simulink model "MicroADPCPU2"  (R2024a)
settings: Solver=FixedStepAuto  StartTime=0.0  StopTime=Inf  RelTol=1e-3  EnableMultiTasking=on
values from neighbouring files (symbols this model uses):
  PI_params = mcb.internal.SetControllerParameters(pmsm,inverter,SI_System,T_pwm,Ts,Ts_speed)    [Para_Motor_Micro.m]
  Ts = T_pwm    (= 3e-05)    [Para_Motor_Micro.m]
  Ts_speed = 10*1*Ts    (= 0.0003)    [Para_Motor_Micro.m]
undefined symbols (not defined in the file or in its folder): C28x, CPU1, CPU2, DiscIntNeverNeededParam
libraries: c2837xDlib x6, mcbcontrolslib x2, c280xlib x2, c2000lib x1, slpidlib x1, svdutilitieslib x1, simulink x1
settings Model: ExtModeTrigDuration=8  Creator=axel_  LastModifiedBy=axel_
settings SolverCC: AutoInsertRateTranBlk=on
settings OptimizationCC: DefaultParameterBehavior=Inlined  DefaultUnderspecifiedDataType=single  EnhancedBackFolding=on  PassReuseOutputArgsAs=Individual arguments  MaxStackSize=1024  OptimizeBlockOrder=speed  DifferentSizesBufferReuse=on  OptimizationCustomize=off  DenormalBehavior=FlushToZero  EfficientTunableParamExpr=on
settings DebuggingCC: MultiTaskDSMMsg=none  ParameterPrecisionLossMsg=none  ParameterTunabilityLossMsg=error
settings HardwareCC: ProdBitPerChar=16  ProdBitPerInt=16  ProdBitPerPointer=32  ProdBitPerSizeT=32  ProdBitPerPtrDiffT=32  ProdLargestAtomicInteger=Integer  ProdLargestAtomicFloat=None  ProdWordSize=16  ProdLongLongMode=on  ProdHWDeviceType=Texas Instruments->C2000
settings ModelReferenceCC: ModelReferenceNumInstancesAllowed=Single
settings SFSimCC: MATLABDynamicMemAlloc=off
settings RTWCC: Description=Embedded Coder  SystemTargetFile=ert.tlc  HardwareBoard=TI Delfino F2837xD  TemplateMakefile=ert_default_tmf  Toolchain=Texas Instruments Code Composer Studio (C2000)  CodeProfilingSaveOptions=MetricsOnly  GPUComputeCapability=3.5
settings CodeAppCC: ForceParamTrailComments=on  IgnoreCustomStorageClasses=off  OperatorAnnotations=on  SimulinkDataObjDesc=on  SFDataObjDesc=on  InsertBlockDesc=on
settings ERTTargetCC: CodeReplacementLibrary=TI C28x  ExtModeTransport=4  ExtModeStaticAlloc=on  ExtModeAutomaticAllocSize=off  ExtModeStaticAllocSize=10000  ExtModeMexFile=ext_xcp  ExtModeIntrfLevel=Level2 - Open  InlinedParameterPlacement=NonHierarchical

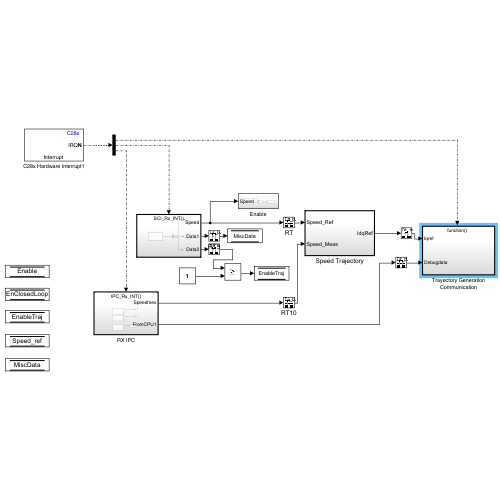
[thumbnail: Simulink's stored preview of the top-level diagram]
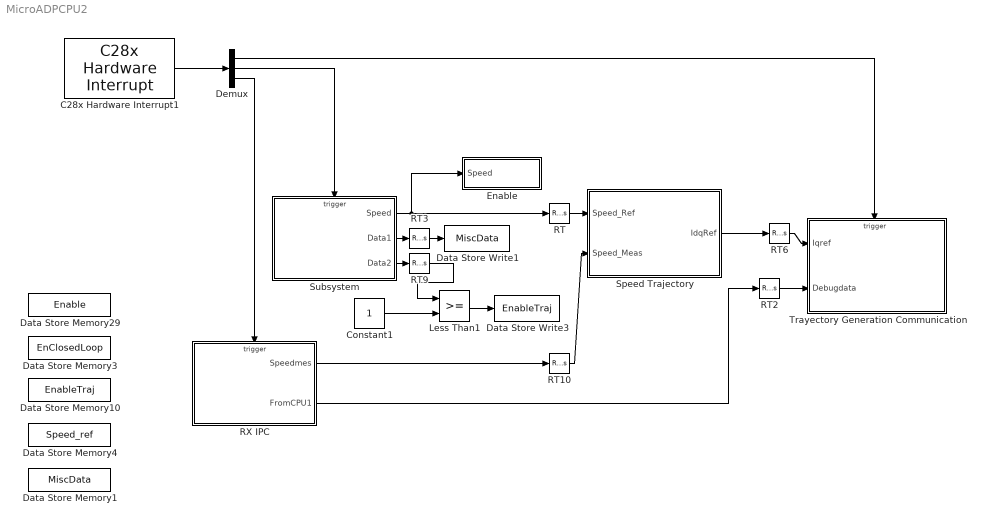
== system MicroADPCPU2 ==
  C28x Hardware Interrupt1 : c2000lib/Scheduling/C28x Hardware Interrupt  irqnumbers=[1 9 1]  pienumbers=[1 1 13]  irqpriorities="[30 50  31]"  irqpreempts=[1 0 1 ]  showinput=off  dspchiptype=C280X
  Constant1 : Constant
  Data Store Memory1 : DataStoreMemory  DataStoreName=MiscData  ShowAdditionalParam=off  OutDataTypeStr=single
  Data Store Memory10 : DataStoreMemory  DataStoreName=EnableTraj  ShowAdditionalParam=off  OutDataTypeStr=boolean
  Data Store Memory29 : DataStoreMemory  DataStoreName=Enable  ShowAdditionalParam=off  OutDataTypeStr=boolean
  Data Store Memory3 : DataStoreMemory  DataStoreName=EnClosedLoop  ShowAdditionalParam=off  OutDataTypeStr=boolean
  Data Store Memory4 : DataStoreMemory  DataStoreName=Speed_ref  InitialValue=20  ShowAdditionalParam=off  OutDataTypeStr=single
  Data Store Write1 : DataStoreWrite  DataStoreName=MiscData  IndexOptions=Index vector (dialog)  Indices=1  OutputSizes=1
  Data Store Write3 : DataStoreWrite  DataStoreName=EnableTraj  IndexOptions=Index vector (dialog)  Indices=1  OutputSizes=1
  Demux : Demux  Outputs=3
  Enable : Subsystem
  Less Than1 : RelationalOperator  OutDataTypeStr=boolean  RndMeth=Simplest  InputSameDT=off
  RT : RateTransition  Deterministic=off  OutPortSampleTime=Ts_speed
  RT10 : RateTransition  Deterministic=off  OutPortSampleTime=Ts_speed
  RT{2..3,6,9} (4 alike) : RateTransition  Deterministic=off
  RX IPC : Subsystem
  Speed Trajectory : Subsystem  TreatAsAtomicUnit=on  SystemSampleTime=Ts_speed
  Subsystem : Subsystem
  Trayectory Generation Communication : Subsystem  TreatAsAtomicUnit=on
  wires:
  C28x Hardware Interrupt1/1 -> Demux/1
  Demux/1 -> Trayectory Generation Communication/Trigger
  Constant1/1 -> Less Than1/2
  Less Than1/1 -> Data Store Write3/1
  Speed Trajectory/1(IdqRef) -> RT6/1
  RT3/1 -> Data Store Write1/1
  RT10/1 -> Speed Trajectory/2(Speed_Meas)
  Subsystem/1(Speed) -> Enable/1(Speed), RT/1
  Subsystem/3(Data2) -> RT9/1
  RT9/1 -> Less Than1/1
  Subsystem/2(Data1) -> RT3/1
  RT/1 -> Speed Trajectory/1(Speed_Ref)
  Demux/2 -> Subsystem/Trigger
  Demux/3 -> RX IPC/Trigger
  RX IPC/1(Speedmes) -> RT10/1
  RT6/1 -> Trayectory Generation Communication/1(Iqref)
  RX IPC/2(FromCPU1) -> RT2/1
  RT2/1 -> Trayectory Generation Communication/2(Debugdata)

== system MicroADPCPU2/Enable ==
  Speed : Inport
  Constant1 : Constant  Value=0
  Data Store Write : DataStoreWrite  DataStoreName=Enable  IndexOptions=Index vector (dialog)  Indices=1  OutputSizes=1
  Less Than : RelationalOperator  Operator=~=  OutDataTypeStr=boolean  RndMeth=Simplest  InputSameDT=off
  wires:
  Less Than/1 -> Data Store Write/1
  Constant1/1 -> Less Than/2
  Speed/1 -> Less Than/1

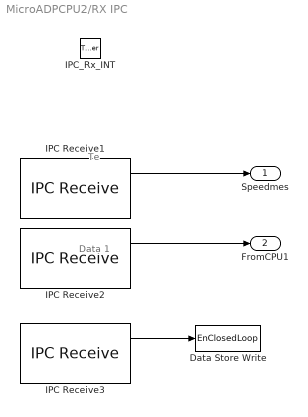
== system MicroADPCPU2/RX IPC ==
  note: Data 1
  note: Te
  IPC_Rx_INT : TriggerPort  TriggerType=function-call  VariantControl=Variant
  Data Store Write : DataStoreWrite  DataStoreName=EnClosedLoop  IndexOptions=Index vector (dialog)  Indices=1  OutputSizes=1
  IPC Receive1 : c2837xDlib/IPC Receive  blkParamProc=F2837x  SelectSource=C28x (CPU1/CPU2)  SelectChannel=0  DataType=single  DataLength=1  EnableBlocking=off  SampleTime=-1
  IPC Receive2 : c2837xDlib/IPC Receive  blkParamProc=F2837x  SelectSource=C28x (CPU1/CPU2)  SelectChannel=1  DataType=single  DataLength=2  EnableBlocking=off  SampleTime=-1
  IPC Receive3 : c2837xDlib/IPC Receive  blkParamProc=F2837x  SelectSource=C28x (CPU1/CPU2)  SelectChannel=4  DataType=boolean  DataLength=1  EnableBlocking=off  SampleTime=-1
  Speedmes : Outport
  FromCPU1 : Outport  Port=2
  wires:
  IPC Receive1/1 -> Speedmes/1
  IPC Receive2/1 -> FromCPU1/1
  IPC Receive3/1 -> Data Store Write/1

== system MicroADPCPU2/Speed Trajectory ==
  Speed_Ref : Inport
  Speed_Meas : Inport  Port=2
  PI_Controller_Speed : Subsystem
  Subsystem : Subsystem
  IdqRef : Outport  VectorParamsAs1DForOutWhenUnconnected=off
  wires:
  Speed_Meas/1 -> PI_Controller_Speed/2(N_fb), Subsystem/2(Speed_Ref_Open)  "Speed_fb"
  Speed_Ref/1 -> Subsystem/1(Speed_Ref_In)
  Subsystem/1(Speed_Ref_PU) -> IdqRef/1, PI_Controller_Speed/1(N_ref)  "Speed_Ref"

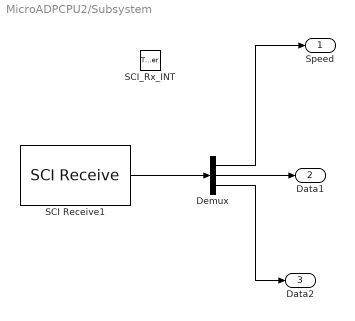
== system MicroADPCPU2/Subsystem ==
  SCI_Rx_INT : TriggerPort  TriggerType=function-call  VariantControl=Variant
  Demux : Demux  Outputs=3
  SCI Receive1 : c280xlib/SCI Receive  sciModule=A  dataHead=''  headerCheckMaxCount=16  dataTail=''  dataType=single  dataLenOptions=Length via dialog  dataDim=3  maxDataLength=1  initValue=0  errOption=Output the last received value  errValue=0  sampleTime=-1  blockingMode=on  timeOut=0.00875  outputStatus=off
  Speed : Outport
  Data1 : Outport  Port=2
  Data2 : Outport  Port=3
  wires:
  Demux/2 -> Data1/1
  SCI Receive1/1 -> Demux/1
  Demux/1 -> Speed/1
  Demux/3 -> Data2/1

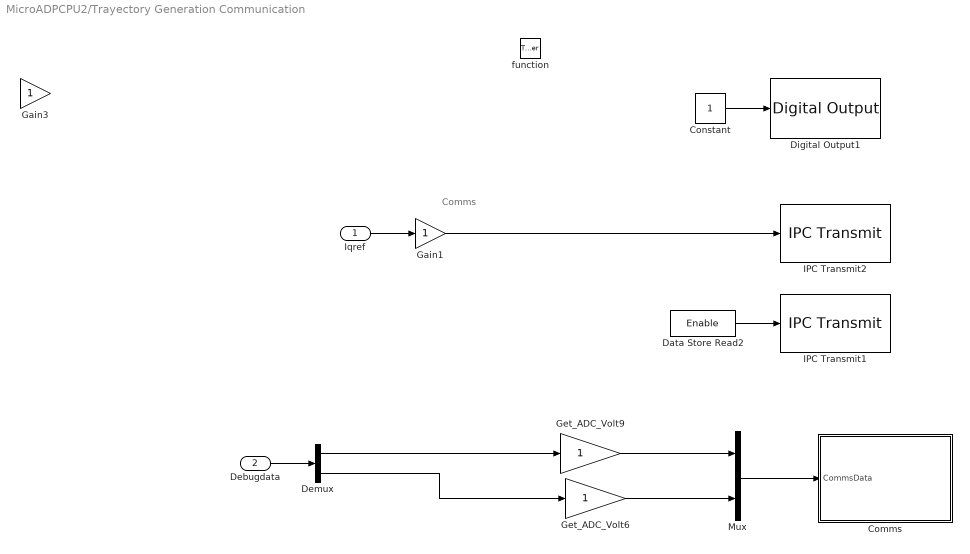
== system MicroADPCPU2/Trayectory Generation Communication ==
  note: Comms
  Iqref : Inport
  Debugdata : Inport  Port=2
  function : TriggerPort  TriggerType=function-call  VariantControl=Variant  OutputDataType=int8
  Comms : Subsystem  SystemSampleTime=5e-5
  Constant : Constant
  Data Store Read2 : DataStoreRead  DataStoreName=Enable  IndexOptions=Index vector (dialog)  Indices=1  OutputSizes=1
  Demux : Demux  Outputs=2
  Digital Output1 : c2837xDlib/Digital Output  GPIO_Number=GPIO16~GPIO23  GPIO_Bit0=off  GPIO_BIT0_Toggle=on  GPIO_Bit1=off  GPIO_BIT1_Toggle=off  GPIO_Bit2=off  GPIO_BIT2_Toggle=off  GPIO_Bit3=off  GPIO_BIT3_Toggle=off  GPIO_Bit4=off  GPIO_BIT4_Toggle=off  GPIO_Bit5=off  GPIO_BIT5_Toggle=off  GPIO_Bit6=on  GPIO_BIT6_Toggle=on  GPIO_Bit7=off  GPIO_BIT7_Toggle=off
  Gain1 : Gain  OutDataTypeStr=single
  Gain3 : Gain  OutDataTypeStr=single
  Get_ADC_Volt6 : Gain  OutDataTypeStr=single  RndMeth=Simplest
  Get_ADC_Volt9 : Gain  OutDataTypeStr=single  RndMeth=Simplest
  IPC Transmit1 : c2837xDlib/IPC Transmit  blkParamProc=F2837x  SelectDestination=C28x (CPU1/CPU2)  SelectChannel=3  EnableBlocking=off
  IPC Transmit2 : c2837xDlib/IPC Transmit  blkParamProc=F2837x  SelectDestination=C28x (CPU1/CPU2)  SelectChannel=2  EnableBlocking=off
  Mux : Mux  Inputs=2
  wires:
  Get_ADC_Volt9/1 -> Mux/1
  Get_ADC_Volt6/1 -> Mux/2
  Mux/1 -> Comms/1(CommsData)
  Data Store Read2/1 -> IPC Transmit1/1
  Iqref/1 -> Gain1/1
  Debugdata/1 -> Demux/1
  Gain1/1 -> IPC Transmit2/1
  Constant/1 -> Digital Output1/1
  Demux/1 -> Get_ADC_Volt9/1
  Demux/2 -> Get_ADC_Volt6/1

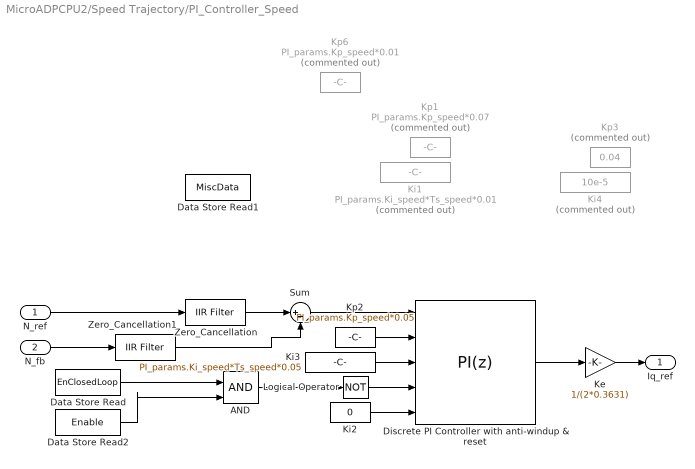
== system MicroADPCPU2/Speed Trajectory/PI_Controller_Speed ==
  N_ref : Inport
  N_fb : Inport  Port=2
  AND : Logic  IconShape=distinctive  AllPortsSameDT=off  OutDataTypeStr=boolean
  Data Store Read : DataStoreRead  DataStoreName=EnClosedLoop  IndexOptions=Index vector (dialog)  Indices=1  OutputSizes=1
  Data Store Read1 : DataStoreRead  DataStoreName=MiscData  IndexOptions=Index vector (dialog)  Indices=1  OutputSizes=1
  Data Store Read2 : DataStoreRead  DataStoreName=Enable  IndexOptions=Index vector (dialog)  Indices=1  OutputSizes=1
  Discrete PI Controller with anti-windup & reset : slpidlib/PID Controller  Controller=PI  Form=Parallel  TimeDomain=Discrete-time  UseExternalTs=off  SampleTime=-1  IntegratorMethod=Forward Euler  FilterMethod=Forward Euler  ControllerParametersSource=external  P=1  I=1  UseKiTs=on  D=0  UseExternalDerivativeSource=off  N=100  UseFilter=on  TunerSelectOption=Transfer Function Based (PID Tuner App)  InitialConditionSource=external  InitialConditionForIntegrator=0  InitialConditionForFilter=0  DifferentiatorICPrevScaledInput=0  ExternalReset=level  TrackingMode=off  Kt=1  LimitOutput=on  SatLimitsSource=internal  UpperSaturationLimit=3.5  LowerSaturationLimit=-3.5  LinearizeAsGain=on  AntiWindupMode=clamping  Kb=1  LimitIntegrator=off  UpperIntegratorSaturationLimit=inf  LowerIntegratorSaturationLimit=-inf  RndMeth=Simplest  POutMin=[]  POutMax=[]  IOutMin=[]  IOutMax=[]  DOutMin=[]  DOutMax=[]  NOutMin=[]  NOutMax=[]  SumOutMin=[]  SumOutMax=[]  SaturationOutDataTypeStr=Inherit: Inherit via back propagation  SaturationOutMin=[]  SaturationOutMax=[]  PParamMin=[]  PParamMax=[]  IParamMin=[]  IParamMax=[]  DParamMin=[]  DParamMax=[]  NParamMin=[]  NParamMax=[]  KbParamMin=[]  KbParamMax=[]  KtParamMin=[]  KtParamMax=[]  KbOutMin=[]  KbOutMax=[]  KtOutMin=[]  KtOutMax=[]  IntegratorOutMin=[]  IntegratorOutMax=[]  FilterOutMin=[]  FilterOutMax=[]  SumI1OutMin=[]  SumI1OutMax=[]  SumI2OutMin=[]  SumI2OutMax=[]  SumI3OutMin=[]  SumI3OutMax=[]  SumI4OutMin=[]  SumI4OutMax=[]  SumDOutMin=[]  SumDOutMax=[]  DifferentiatorOutMin=[]  DifferentiatorOutMax=[]  FilterDiffOutCoefMin=[]  FilterDiffOutCoefMax=[]  ReciprocalOutMin=[]  ReciprocalOutMax=[]  SumDenOutMin=[]  SumDenOutMax=[]  SumNumOutMin=[]  SumNumOutMax=[]  DivideOutMin=[]  DivideOutMax=[]  UdiffTsProdOutMin=[]  UdiffTsProdOutMax=[]  NTsProdOutMin=[]  NTsProdOutMax=[]  UintegralTsProdOutMin=[]  UintegralTsProdOutMax=[]  UngainTsProdOutMin=[]  UngainTsProdOutMax=[]  ClampingZeroOutDataTypeStr=Inherit: Inherit via back propagation  ClampingZeroOutMin=[]  ClampingZeroOutMax=[]  FilterDenConstantOutDataTypeStr=Inherit: Inherit via back propagation  FilterDenConstantOutMin=[]  FilterDenConstantOutMax=[]  PCopyOutDataTypeStr=Inherit: Inherit via back propagation  PCopyOutMin=[]  PCopyOutMax=[]  NCopyOutDataTypeStr=Inherit: Inherit via back propagation  NCopyOutMin=[]  NCopyOutMax=[]  IntegratorContinuousStateAttributes=''  IntegratorStateMustResolveToSignalObject=off  IntegratorRTWStateStorageClass=Auto  FilterContinuousStateAttributes=''  FilterStateMustResolveToSignalObject=off  FilterRTWStateStorageClass=Auto  ParallelPVariant=ExternalParameters  IdealPVariant=Disabled  IVariant=ExternalParameters  DVariant=Disabled  IntegratorVariant=Discrete  SatVariant=Enabled  AWVariant=DiscClampingParallel  PCopyVariant=Disabled  TRVariant=Disabled  FdbkBlocksVariant=Forward  IdealPFdbkVariant=Disabled  SatFdbkVariant=Disabled  DerivativeFilterVariant=Disabled  NVariant=Disabled  NCopyVariant=Disabled_SignalSpec  FilterICVariant=Disabled  IntegratorICVariant=ExternalICs  ExternalResetVariant=ExternalReset  TRSumVariant=Passthrough  SumFdbkVariant=Disabled  SumVariant=Sum_PI  TsampFilterVariant=InternalTs  TsampNgainVariant=Passthrough  TsampIntegralVariant=Disabled_SignalSpec  ExternalSaturationOutDataTypeStr=Inherit: Same as second input  DerivativeSourceVariant=Disabled
      settings: LibrarySourceBlock=mcbcontrolslib/PI Controller
  Ke : Gain  Gain=1/(2*0.3631)  OutDataTypeStr=single
  Ki1 : Constant  Commented=on  Value=PI_params.Ki_speed*Ts_speed*0.01  OutDataTypeStr=double  SampleTime=-1
  Ki2 : Constant  Value=0  OutDataTypeStr=dataType  SampleTime=-1
  Ki3 : Constant  Value=PI_params.Ki_speed*Ts_speed*0.05  OutDataTypeStr=double  SampleTime=-1
  Ki4 : Constant  Commented=on  Value=10e-5  OutDataTypeStr=double  SampleTime=-1
  Kp1 : Constant  Commented=on  Value=PI_params.Kp_speed*0.07  OutDataTypeStr=double  SampleTime=-1
  Kp2 : Constant  Value=PI_params.Kp_speed*0.05  OutDataTypeStr=double  SampleTime=-1
  Kp3 : Constant  Commented=on  Value=0.04  OutDataTypeStr=double  SampleTime=-1
  Kp6 : Constant  Commented=on  Value=PI_params.Kp_speed*0.01  OutDataTypeStr=double  SampleTime=-1
  Logical Operator : Logic  Operator=NOT  IconShape=distinctive  AllPortsSameDT=off  OutDataTypeStr=boolean
  Sum : Sum  Inputs=|+-  OutDataTypeStr=Inherit: Same as first input
  Zero_Cancellation : mcbcontrolslib/IIR Filter  VariantControl=Low Pass Filter  VariantSelect=Low-pass  FilterConstantInputType=Specify via dialog  Filter_constant=0.01*(Ts_speed/Ts)  advancedSettings=off  Ts=50e-6  cutOff_freq=353.6777
  Zero_Cancellation1 : mcbcontrolslib/IIR Filter  VariantControl=Low Pass Filter  VariantSelect=Low-pass  FilterConstantInputType=Specify via dialog  Filter_constant=0.01*(Ts_speed/Ts)  advancedSettings=off  Ts=50e-6  cutOff_freq=353.6777
  Iq_ref : Outport  VectorParamsAs1DForOutWhenUnconnected=off
  wires:
  Discrete PI Controller with anti-windup & reset/1 -> Ke/1
  Sum/1 -> Discrete PI Controller with anti-windup & reset/1
  Logical Operator/1 -> Discrete PI Controller with anti-windup & reset/4
  Ki2/1 -> Discrete PI Controller with anti-windup & reset/5
  AND/1 -> Logical Operator/1
  N_ref/1 -> Zero_Cancellation/1
  N_fb/1 -> Zero_Cancellation1/1
  Zero_Cancellation/1 -> Sum/1
  Data Store Read/1 -> AND/1
  Data Store Read2/1 -> AND/2
  Ki3/1 -> Discrete PI Controller with anti-windup & reset/3
  Kp2/1 -> Discrete PI Controller with anti-windup & reset/2
  Zero_Cancellation1/1 -> Sum/2
  Ke/1 -> Iq_ref/1

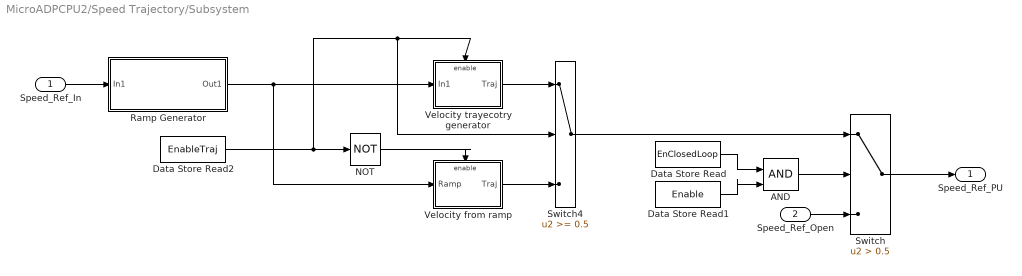
== system MicroADPCPU2/Speed Trajectory/Subsystem ==
  Speed_Ref_In : Inport
  Speed_Ref_Open : Inport  Port=2
  AND : Logic  IconShape=distinctive  AllPortsSameDT=off  OutDataTypeStr=boolean
  Data Store Read : DataStoreRead  DataStoreName=EnClosedLoop  IndexOptions=Index vector (dialog)  Indices=1  OutputSizes=1
  Data Store Read1 : DataStoreRead  DataStoreName=Enable  IndexOptions=Index vector (dialog)  Indices=1  OutputSizes=1
  Data Store Read2 : DataStoreRead  DataStoreName=EnableTraj  IndexOptions=Index vector (dialog)  Indices=1  OutputSizes=1
  NOT : Logic  Operator=NOT  IconShape=distinctive  AllPortsSameDT=off  OutDataTypeStr=boolean
  Ramp Generator : Subsystem
  Switch : Switch  Criteria=u2 > Threshold  Threshold=0.5  SaturateOnIntegerOverflow=off  InputSameDT=off
  Switch4 : Switch  Threshold=0.5  OutDataTypeStr=Inherit: Inherit via back propagation  RndMeth=Simplest  SaturateOnIntegerOverflow=off  InputSameDT=off
  Velocity from ramp : Subsystem
  Velocity trayecotry generator : Subsystem
  Speed_Ref_PU : Outport
  wires:
  Switch/1 -> Speed_Ref_PU/1
  Speed_Ref_Open/1 -> Switch/3
  AND/1 -> Switch/2
  Data Store Read/1 -> AND/1
  Data Store Read1/1 -> AND/2
  Data Store Read2/1 -> Switch4/2, Velocity trayecotry generator/Enable, NOT/1
  Velocity from ramp/1(Traj) -> Switch4/3
  NOT/1 -> Velocity from ramp/Enable
  Velocity trayecotry generator/1(Traj) -> Switch4/1
  Switch4/1 -> Switch/1
  Ramp Generator/1(Out1) -> Velocity trayecotry generator/1(In1), Velocity from ramp/1(Ramp)
  Speed_Ref_In/1 -> Ramp Generator/1(In1)

== system MicroADPCPU2/Trayectory Generation Communication/Comms ==
  CommsData : Inport
  SCI (Serial Comunication) : Subsystem
  Selector : Selector  InputPortWidth=2  IndexOptions=Index vector (port)  Indices=[1 3]  OutputSizes=1
  speed_control : Constant  Value=[1 2]  OutDataTypeStr=uint16  SampleTime=-1
  wires:
  Selector/1 -> SCI (Serial Comunication)/1(In1)
  CommsData/1 -> Selector/1
  speed_control/1 -> Selector/2

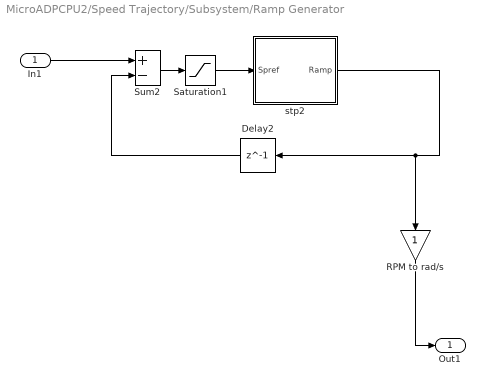
== system MicroADPCPU2/Speed Trajectory/Subsystem/Ramp Generator ==
  In1 : Inport
  Delay2 : Delay  DelayLength=1
  RPM to rad/s : Gain  OutDataTypeStr=single  RndMeth=Simplest
  Saturation1 : Saturate  UpperLimit=2.5e-3  LowerLimit=-2.5e-3  OutDataTypeStr=double
  Sum2 : Sum  Inputs=+-
  stp2 : MATLAB Function  TreatAsAtomicUnit=on
  Out1 : Outport
  wires:
  Saturation1/1 -> stp2/1(Spref)
  stp2/1(Ramp) -> RPM to rad/s/1, Delay2/1
  Delay2/1 -> Sum2/2
  RPM to rad/s/1 -> Out1/1
  Sum2/1 -> Saturation1/1
  In1/1 -> Sum2/1

== system MicroADPCPU2/Speed Trajectory/Subsystem/Velocity from ramp ==
  Ramp : Inport
  Enable : EnablePort  StatesWhenEnabling=reset
  Traj : Outport  VectorParamsAs1DForOutWhenUnconnected=off
  wires:
  Ramp/1 -> Traj/1

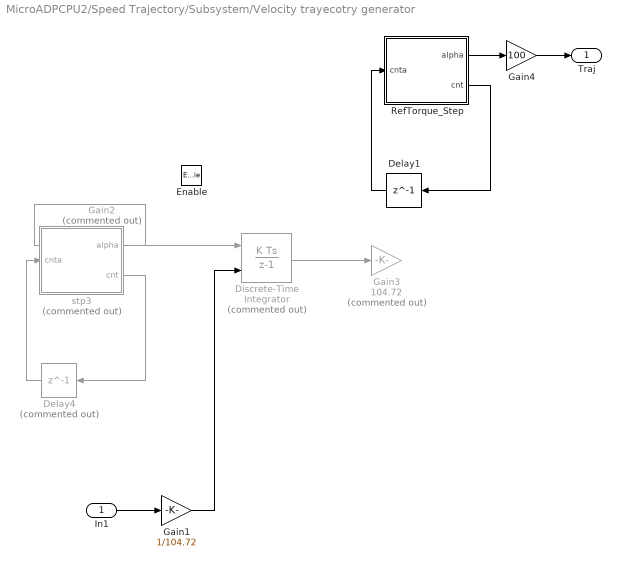
== system MicroADPCPU2/Speed Trajectory/Subsystem/Velocity trayecotry generator ==
  In1 : Inport
  Enable : EnablePort  StatesWhenEnabling=reset
  Delay1 : Delay  DelayLength=1
  Delay4 : Delay  Commented=on  DelayLength=1
  Discrete-Time Integrator : DiscreteIntegrator  Commented=on  InitialConditionSource=external  InitialCondition=0.47746371  SampleTime=-1  ICPrevOutput=DiscIntNeverNeededParam  ICPrevScaledInput=DiscIntNeverNeededParam
  Gain1 : Gain  Gain=1/104.72  OutDataTypeStr=single
  Gain2 : Gain  Commented=on  OutDataTypeStr=single
  Gain3 : Gain  Commented=on  Gain=104.72  OutDataTypeStr=single
  Gain4 : Gain  Gain=100  OutDataTypeStr=single
  RefTorque_Step : MATLAB Function  TreatAsAtomicUnit=on
  stp3 : MATLAB Function  Commented=on  TreatAsAtomicUnit=on
  Traj : Outport  VectorParamsAs1DForOutWhenUnconnected=off
  wires:
  Discrete-Time Integrator/1 -> Gain3/1
  Delay4/1 -> stp3/1(cnta)
  stp3/2(cnt) -> Delay4/1
  stp3/1(alpha) -> Gain2/1
  In1/1 -> Gain1/1
  Gain1/1 -> Discrete-Time Integrator/2
  Gain2/1 -> Discrete-Time Integrator/1
  RefTorque_Step/1(alpha) -> Gain4/1
  RefTorque_Step/2(cnt) -> Delay1/1
  Delay1/1 -> RefTorque_Step/1(cnta)
  Gain4/1 -> Traj/1

== system MicroADPCPU2/Trayectory Generation Communication/Comms/SCI (Serial Comunication) ==
  In1 : Inport
  Byte Pack : svdutilitieslib/Byte Pack  maskPackedDataType=uint32  datatypes={'single'}  byteAlign=4  blockPlatform=tic2000
  Data_Logging : Subsystem
  Demux2 : Demux  Outputs=2
  While Iterator Subsystem : Subsystem  TreatAsAtomicUnit=on
  wires:
  Demux2/2 -> While Iterator Subsystem/2(Iteration)  "SCI_Tx_Iteration"
  Demux2/1 -> While Iterator Subsystem/1(Data)  "SCI_Tx_Data"
  In1/1 -> Byte Pack/1
  Data_Logging/1(SCI_Tx) -> Demux2/1
  Byte Pack/1 -> Data_Logging/1(Data_Log)

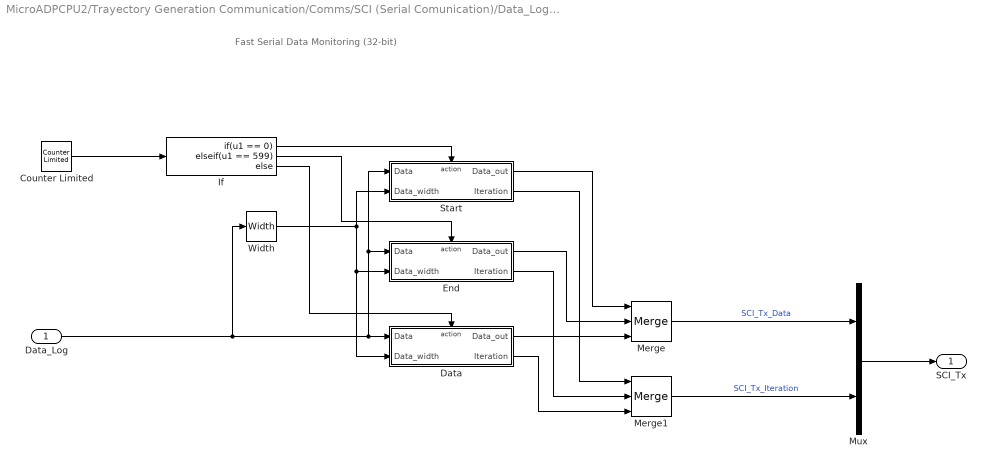
== system MicroADPCPU2/Trayectory Generation Communication/Comms/SCI (Serial Comunication)/Data_Logging ==
  note: Fast Serial Data Monitoring (32-bit)
  Data_Log : Inport
  Counter Limited : simulink/Sources/Counter Limited  uplimit=600-1  tsamp=-1
  Data : Subsystem  TreatAsAtomicUnit=on
  End : Subsystem  TreatAsAtomicUnit=on
  If : If  IfExpression=u1 == 0  ElseIfExpressions=u1 == 599
  Merge : Merge  Inputs=3
  Merge1 : Merge  Inputs=3
  Mux : Mux  Inputs=2
  Start : Subsystem  TreatAsAtomicUnit=on
  Width : Width  OutDataTypeMode=All ports same datatype  DataType=uint16
  SCI_Tx : Outport
  wires:
  If/3 -> Data/Action
  Data/1(Data_out) -> Merge/3
  Width/1 -> Data/2(Data_width), End/2(Data_width), Start/2(Data_width)
  Merge/1 -> Mux/1  "SCI_Tx_Data"
  Counter Limited/1 -> If/1
  Start/2(Iteration) -> Merge1/1
  Start/1(Data_out) -> Merge/1
  If/2 -> End/Action
  Merge1/1 -> Mux/2  "SCI_Tx_Iteration"
  If/1 -> Start/Action
  End/1(Data_out) -> Merge/2
  End/2(Iteration) -> Merge1/2
  Data/2(Iteration) -> Merge1/3
  Mux/1 -> SCI_Tx/1
  Data_Log/1 -> Width/1, Start/1(Data), End/1(Data), Data/1(Data)

== system MicroADPCPU2/Trayectory Generation Communication/Comms/SCI (Serial Comunication)/While Iterator Subsystem ==
  Data : Inport
  Iteration : Inport  Port=2
  Add : Sum  Inputs=+-  OutDataTypeStr=Inherit: Same as first input
  Index Vector : MultiPortSwitch  Inputs=1  SaturateOnIntegerOverflow=off  InputSameDT=off
  SCI Transmit : c280xlib/SCI Transmit  sciModule=A  dataHead=''  dataTail=''  frameSize=1  blockingMode=on  outputStatus=off
  While Iterator : WhileIterator  MaxIters=-1  WhileBlockType=do-while  ShowIterationPort=on  OutputDataType=int16
  wires:
  While Iterator/1 -> Add/2, Index Vector/1
  Data/1 -> Index Vector/2
  Index Vector/1 -> SCI Transmit/1
  Add/1 -> While Iterator/1
  Iteration/1 -> Add/1

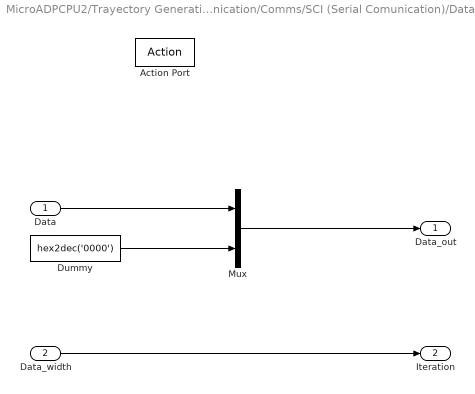
== system MicroADPCPU2/Trayectory Generation Communication/Comms/SCI (Serial Comunication)/Data_Logging/Data ==
  Data : Inport
  Data_width : Inport  Port=2
  Action Port : ActionPort  ActionPortLabel=else
  Dummy : Constant  Value=hex2dec('0000')  OutDataTypeStr=uint32
  Mux : Mux  Inputs=2
  Data_out : Outport  VectorParamsAs1DForOutWhenUnconnected=off
  Iteration : Outport  Port=2  VectorParamsAs1DForOutWhenUnconnected=off
  wires:
  Data_width/1 -> Iteration/1
  Data/1 -> Mux/1
  Dummy/1 -> Mux/2
  Mux/1 -> Data_out/1

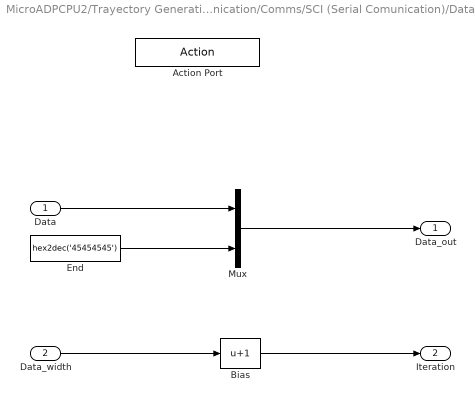
== system MicroADPCPU2/Trayectory Generation Communication/Comms/SCI (Serial Comunication)/Data_Logging/End ==
  Data : Inport
  Data_width : Inport  Port=2
  Action Port : ActionPort  ActionPortLabel=elseif(u1 == 599)
  Bias : Bias  Bias=1  SaturateOnIntegerOverflow=off
  End : Constant  Value=hex2dec('45454545')  OutDataTypeStr=uint32
  Mux : Mux  Inputs=2
  Data_out : Outport  VectorParamsAs1DForOutWhenUnconnected=off
  Iteration : Outport  Port=2  VectorParamsAs1DForOutWhenUnconnected=off
  wires:
  Data/1 -> Mux/1
  Data_width/1 -> Bias/1
  Bias/1 -> Iteration/1
  End/1 -> Mux/2
  Mux/1 -> Data_out/1

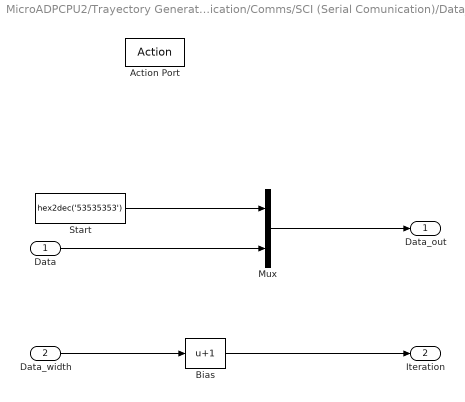
== system MicroADPCPU2/Trayectory Generation Communication/Comms/SCI (Serial Comunication)/Data_Logging/Start ==
  Data : Inport
  Data_width : Inport  Port=2
  Action Port : ActionPort  ActionPortLabel=if(u1 == 0)
  Bias : Bias  Bias=1  SaturateOnIntegerOverflow=off
  Mux : Mux  Inputs=2
  Start : Constant  Value=hex2dec('53535353')  OutDataTypeStr=uint32
  Data_out : Outport  VectorParamsAs1DForOutWhenUnconnected=off
  Iteration : Outport  Port=2  VectorParamsAs1DForOutWhenUnconnected=off
  wires:
  Data/1 -> Mux/2
  Data_width/1 -> Bias/1
  Bias/1 -> Iteration/1
  Start/1 -> Mux/1
  Mux/1 -> Data_out/1

== matlab function MicroADPCPU2/Speed Trajectory/Subsystem/Velocity trayecotry generator/RefTorque_Step ==
  settings: updateMethod=DISCRETE
  data: cnta input; alpha output; cnt output
function [alpha,cnt]        = fcn(cnta)
cnt=1+cnta;
t=(5e-4)*cnt;
if t<5
 alpha=0.15  ;
elseif t<=5.3
   alpha=0.20; 
      elseif t<=5.5
           alpha=0.18; 
   % elseif t<=5.7
   %  alpha=0.21; 
        
   else      
    alpha=0.14  ;
    
end

== matlab function MicroADPCPU2/Speed Trajectory/Subsystem/Velocity trayecotry generator/stp3 ==
  settings: updateMethod=DISCRETE
  data: cnta input; alpha output; cnt output
function [alpha,cnt]        = fcn(cnta)
cnt=1+cnta;
t=(2e-4)*cnt;
if t<2
 alpha=0  ;
elseif t<=3.9
   alpha=0.5; 
      elseif t<=5.8
           alpha=0; 
   elseif t<=6
    alpha=0; 
         elseif t<=7
    alpha=0;
 elseif t<=8
  alpha=-(0.3)*t +2.1;   
   elseif t<=9
  alpha=(0.3)*t -2.7 ;  
  elseif t<=12
    alpha=0;
    elseif t<=13
  alpha=-0.3;
   elseif t<=14
  alpha=0 ; 
    elseif t<=17
    alpha=0;
    
       elseif t<=18
    alpha=(-.2)*t +3.4;
    
           elseif t<=19
    alpha=(+.2)*t -3.8 ;
    
 else      
    alpha=0  ;
    
end

== matlab function MicroADPCPU2/Speed Trajectory/Subsystem/Ramp Generator/stp2 ==
  settings: updateMethod=DISCRETE
  data: Spref input; Ramp output
function Ramp        = fcn(Spref)
persistent Speedref
    if isempty(Speedref)
        Speedref = 0;
    end
     
Speedref=Spref+Speedref;
Ramp=Speedref;
    
end
